simulink subsystem "PvtSubSys_HMI"  (R2020b)
settings: Solver=VariableStepAuto  StartTime=0.0  StopTime=10.0  RelTol=1e-3
undefined symbols (not defined in the file): P_HMI_LDW_LKAWarnTime, P_HMI_ObjectTypeFilter, P_HMI_WarnFormLDWReq
libraries: simulink x212, TrueDurationTime x6
(part 6 of 8)

== system PvtSubSys_HMI/HMI2.12/IFC_Signal1/Subsystem30 ==
  note: When the vehicle stops, stop updating
  note: 存在一帧丢失状况
  standstill : Inport
  in : Inport  Port=2
  Compare To Constant10 : simulink/Logic and Bit Operations/Compare To Constant  relop===  const=1  OutDataTypeStr=boolean
  Compare To Constant9 : simulink/Logic and Bit Operations/Compare To Constant  relop===  const=0  OutDataTypeStr=boolean
  Logical Operator8 : Logic  AllPortsSameDT=off  OutDataTypeStr=boolean
  MATLAB Function1 : MATLAB Function  TreatAsAtomicUnit=on
  Unit Delay : UnitDelay  SampleTime=-1  HasFrameUpgradeWarning=on
  Unit Delay3 : UnitDelay  SampleTime=-1  HasFrameUpgradeWarning=on
  out : Outport
  wires:
  Logical Operator8/1 -> MATLAB Function1/3(update)
  standstill/1 -> MATLAB Function1/1(standstill), Compare To Constant10/1, Unit Delay3/1
  Compare To Constant9/1 -> Logical Operator8/1
  in/1 -> MATLAB Function1/2(in)
  MATLAB Function1/2(recorder) -> Unit Delay/1
  Unit Delay3/1 -> Compare To Constant9/1
  Compare To Constant10/1 -> Logical Operator8/2
  Unit Delay/1 -> MATLAB Function1/4(inrecorder)
  MATLAB Function1/1(out) -> out/1

== system PvtSubSys_HMI/HMI2.12/IFC_Signal1/Subsystem31 ==
  note: 存在一帧丢失状况
  note: When the vehicle stops, stop updating
  standstill : Inport
  in : Inport  Port=2
  Compare To Constant10 : simulink/Logic and Bit Operations/Compare To Constant  relop===  const=1  OutDataTypeStr=boolean
  Compare To Constant9 : simulink/Logic and Bit Operations/Compare To Constant  relop===  const=0  OutDataTypeStr=boolean
  Logical Operator8 : Logic  AllPortsSameDT=off  OutDataTypeStr=boolean
  MATLAB Function1 : MATLAB Function  TreatAsAtomicUnit=on
  Unit Delay : UnitDelay  SampleTime=-1  HasFrameUpgradeWarning=on
  Unit Delay3 : UnitDelay  SampleTime=-1  HasFrameUpgradeWarning=on
  out : Outport
  wires:
  MATLAB Function1/1(out) -> out/1
  Unit Delay/1 -> MATLAB Function1/4(inrecorder)
  Compare To Constant10/1 -> Logical Operator8/2
  Unit Delay3/1 -> Compare To Constant9/1
  MATLAB Function1/2(recorder) -> Unit Delay/1
  in/1 -> MATLAB Function1/2(in)
  Compare To Constant9/1 -> Logical Operator8/1
  standstill/1 -> Unit Delay3/1, Compare To Constant10/1, MATLAB Function1/1(standstill)
  Logical Operator8/1 -> MATLAB Function1/3(update)

== system PvtSubSys_HMI/HMI2.12/IFC_Signal1/Subsystem32 ==
  note: When the vehicle stops, stop updating
  note: 存在一帧丢失状况
  standstill : Inport
  in : Inport  Port=2
  Compare To Constant10 : simulink/Logic and Bit Operations/Compare To Constant  relop===  const=1  OutDataTypeStr=boolean
  Compare To Constant9 : simulink/Logic and Bit Operations/Compare To Constant  relop===  const=0  OutDataTypeStr=boolean
  Logical Operator8 : Logic  AllPortsSameDT=off  OutDataTypeStr=boolean
  MATLAB Function1 : MATLAB Function  TreatAsAtomicUnit=on
  Unit Delay : UnitDelay  SampleTime=-1  HasFrameUpgradeWarning=on
  Unit Delay3 : UnitDelay  SampleTime=-1  HasFrameUpgradeWarning=on
  out : Outport
  wires:
  Logical Operator8/1 -> MATLAB Function1/3(update)
  standstill/1 -> MATLAB Function1/1(standstill), Compare To Constant10/1, Unit Delay3/1
  Compare To Constant9/1 -> Logical Operator8/1
  in/1 -> MATLAB Function1/2(in)
  MATLAB Function1/2(recorder) -> Unit Delay/1
  Unit Delay3/1 -> Compare To Constant9/1
  Compare To Constant10/1 -> Logical Operator8/2
  Unit Delay/1 -> MATLAB Function1/4(inrecorder)
  MATLAB Function1/1(out) -> out/1

== system PvtSubSys_HMI/HMI2.12/IFC_Signal1/Subsystem33 ==
  note: 存在一帧丢失状况
  note: When the vehicle stops, stop updating
  standstill : Inport
  in : Inport  Port=2
  Compare To Constant10 : simulink/Logic and Bit Operations/Compare To Constant  relop===  const=1  OutDataTypeStr=boolean
  Compare To Constant9 : simulink/Logic and Bit Operations/Compare To Constant  relop===  const=0  OutDataTypeStr=boolean
  Logical Operator8 : Logic  AllPortsSameDT=off  OutDataTypeStr=boolean
  MATLAB Function1 : MATLAB Function  TreatAsAtomicUnit=on
  Unit Delay : UnitDelay  SampleTime=-1  HasFrameUpgradeWarning=on
  Unit Delay3 : UnitDelay  SampleTime=-1  HasFrameUpgradeWarning=on
  out : Outport
  wires:
  MATLAB Function1/1(out) -> out/1
  Unit Delay/1 -> MATLAB Function1/4(inrecorder)
  Compare To Constant10/1 -> Logical Operator8/2
  Unit Delay3/1 -> Compare To Constant9/1
  MATLAB Function1/2(recorder) -> Unit Delay/1
  in/1 -> MATLAB Function1/2(in)
  Compare To Constant9/1 -> Logical Operator8/1
  standstill/1 -> Unit Delay3/1, Compare To Constant10/1, MATLAB Function1/1(standstill)
  Logical Operator8/1 -> MATLAB Function1/3(update)

== system PvtSubSys_HMI/HMI2.12/IFC_Signal1/Subsystem34 ==
  note: When the vehicle stops, stop updating
  note: 存在一帧丢失状况
  standstill : Inport
  in : Inport  Port=2
  Compare To Constant10 : simulink/Logic and Bit Operations/Compare To Constant  relop===  const=1  OutDataTypeStr=boolean
  Compare To Constant9 : simulink/Logic and Bit Operations/Compare To Constant  relop===  const=0  OutDataTypeStr=boolean
  Logical Operator8 : Logic  AllPortsSameDT=off  OutDataTypeStr=boolean
  MATLAB Function1 : MATLAB Function  TreatAsAtomicUnit=on
  Unit Delay : UnitDelay  SampleTime=-1  HasFrameUpgradeWarning=on
  Unit Delay3 : UnitDelay  SampleTime=-1  HasFrameUpgradeWarning=on
  out : Outport
  wires:
  Logical Operator8/1 -> MATLAB Function1/3(update)
  standstill/1 -> MATLAB Function1/1(standstill), Compare To Constant10/1, Unit Delay3/1
  Compare To Constant9/1 -> Logical Operator8/1
  in/1 -> MATLAB Function1/2(in)
  MATLAB Function1/2(recorder) -> Unit Delay/1
  Unit Delay3/1 -> Compare To Constant9/1
  Compare To Constant10/1 -> Logical Operator8/2
  Unit Delay/1 -> MATLAB Function1/4(inrecorder)
  MATLAB Function1/1(out) -> out/1

== system PvtSubSys_HMI/HMI2.12/IFC_Signal1/Subsystem35 ==
  note: When the vehicle stops, stop updating
  note: 存在一帧丢失状况
  standstill : Inport
  in : Inport  Port=2
  Compare To Constant10 : simulink/Logic and Bit Operations/Compare To Constant  relop===  const=1  OutDataTypeStr=boolean
  Compare To Constant9 : simulink/Logic and Bit Operations/Compare To Constant  relop===  const=0  OutDataTypeStr=boolean
  Logical Operator8 : Logic  AllPortsSameDT=off  OutDataTypeStr=boolean
  MATLAB Function1 : MATLAB Function  TreatAsAtomicUnit=on
  Unit Delay : UnitDelay  SampleTime=-1  HasFrameUpgradeWarning=on
  Unit Delay3 : UnitDelay  SampleTime=-1  HasFrameUpgradeWarning=on
  out : Outport
  wires:
  Logical Operator8/1 -> MATLAB Function1/3(update)
  standstill/1 -> MATLAB Function1/1(standstill), Compare To Constant10/1, Unit Delay3/1
  Compare To Constant9/1 -> Logical Operator8/1
  in/1 -> MATLAB Function1/2(in)
  MATLAB Function1/2(recorder) -> Unit Delay/1
  Unit Delay3/1 -> Compare To Constant9/1
  Compare To Constant10/1 -> Logical Operator8/2
  Unit Delay/1 -> MATLAB Function1/4(inrecorder)
  MATLAB Function1/1(out) -> out/1

== system PvtSubSys_HMI/HMI2.12/IFC_Signal1/Subsystem36 ==
  note: 存在一帧丢失状况
  note: When the vehicle stops, stop updating
  standstill : Inport
  in : Inport  Port=2
  Compare To Constant10 : simulink/Logic and Bit Operations/Compare To Constant  relop===  const=1  OutDataTypeStr=boolean
  Compare To Constant9 : simulink/Logic and Bit Operations/Compare To Constant  relop===  const=0  OutDataTypeStr=boolean
  Logical Operator8 : Logic  AllPortsSameDT=off  OutDataTypeStr=boolean
  MATLAB Function1 : MATLAB Function  TreatAsAtomicUnit=on
  Unit Delay : UnitDelay  SampleTime=-1  HasFrameUpgradeWarning=on
  Unit Delay3 : UnitDelay  SampleTime=-1  HasFrameUpgradeWarning=on
  out : Outport
  wires:
  MATLAB Function1/1(out) -> out/1
  Unit Delay/1 -> MATLAB Function1/4(inrecorder)
  Compare To Constant10/1 -> Logical Operator8/2
  Unit Delay3/1 -> Compare To Constant9/1
  MATLAB Function1/2(recorder) -> Unit Delay/1
  in/1 -> MATLAB Function1/2(in)
  Compare To Constant9/1 -> Logical Operator8/1
  standstill/1 -> Unit Delay3/1, Compare To Constant10/1, MATLAB Function1/1(standstill)
  Logical Operator8/1 -> MATLAB Function1/3(update)

== system PvtSubSys_HMI/HMI2.12/IFC_Signal1/Subsystem37 ==
  note: When the vehicle stops, stop updating
  note: 存在一帧丢失状况
  standstill : Inport
  in : Inport  Port=2
  Compare To Constant10 : simulink/Logic and Bit Operations/Compare To Constant  relop===  const=1  OutDataTypeStr=boolean
  Compare To Constant9 : simulink/Logic and Bit Operations/Compare To Constant  relop===  const=0  OutDataTypeStr=boolean
  Logical Operator8 : Logic  AllPortsSameDT=off  OutDataTypeStr=boolean
  MATLAB Function1 : MATLAB Function  TreatAsAtomicUnit=on
  Unit Delay : UnitDelay  SampleTime=-1  HasFrameUpgradeWarning=on
  Unit Delay3 : UnitDelay  SampleTime=-1  HasFrameUpgradeWarning=on
  out : Outport
  wires:
  Logical Operator8/1 -> MATLAB Function1/3(update)
  standstill/1 -> MATLAB Function1/1(standstill), Compare To Constant10/1, Unit Delay3/1
  Compare To Constant9/1 -> Logical Operator8/1
  in/1 -> MATLAB Function1/2(in)
  MATLAB Function1/2(recorder) -> Unit Delay/1
  Unit Delay3/1 -> Compare To Constant9/1
  Compare To Constant10/1 -> Logical Operator8/2
  Unit Delay/1 -> MATLAB Function1/4(inrecorder)
  MATLAB Function1/1(out) -> out/1

== system PvtSubSys_HMI/HMI2.12/IFC_Signal1/Subsystem38 ==
  note: 存在一帧丢失状况
  note: When the vehicle stops, stop updating
  standstill : Inport
  in : Inport  Port=2
  Compare To Constant10 : simulink/Logic and Bit Operations/Compare To Constant  relop===  const=1  OutDataTypeStr=boolean
  Compare To Constant9 : simulink/Logic and Bit Operations/Compare To Constant  relop===  const=0  OutDataTypeStr=boolean
  Logical Operator8 : Logic  AllPortsSameDT=off  OutDataTypeStr=boolean
  MATLAB Function1 : MATLAB Function  TreatAsAtomicUnit=on
  Unit Delay : UnitDelay  SampleTime=-1  HasFrameUpgradeWarning=on
  Unit Delay3 : UnitDelay  SampleTime=-1  HasFrameUpgradeWarning=on
  out : Outport
  wires:
  MATLAB Function1/1(out) -> out/1
  Unit Delay/1 -> MATLAB Function1/4(inrecorder)
  Compare To Constant10/1 -> Logical Operator8/2
  Unit Delay3/1 -> Compare To Constant9/1
  MATLAB Function1/2(recorder) -> Unit Delay/1
  in/1 -> MATLAB Function1/2(in)
  Compare To Constant9/1 -> Logical Operator8/1
  standstill/1 -> Unit Delay3/1, Compare To Constant10/1, MATLAB Function1/1(standstill)
  Logical Operator8/1 -> MATLAB Function1/3(update)

== system PvtSubSys_HMI/HMI2.12/IFC_Signal1/Subsystem39 ==
  note: When the vehicle stops, stop updating
  note: 存在一帧丢失状况
  standstill : Inport
  in : Inport  Port=2
  Compare To Constant10 : simulink/Logic and Bit Operations/Compare To Constant  relop===  const=1  OutDataTypeStr=boolean
  Compare To Constant9 : simulink/Logic and Bit Operations/Compare To Constant  relop===  const=0  OutDataTypeStr=boolean
  Logical Operator8 : Logic  AllPortsSameDT=off  OutDataTypeStr=boolean
  MATLAB Function1 : MATLAB Function  TreatAsAtomicUnit=on
  Unit Delay : UnitDelay  SampleTime=-1  HasFrameUpgradeWarning=on
  Unit Delay3 : UnitDelay  SampleTime=-1  HasFrameUpgradeWarning=on
  out : Outport
  wires:
  Logical Operator8/1 -> MATLAB Function1/3(update)
  standstill/1 -> MATLAB Function1/1(standstill), Compare To Constant10/1, Unit Delay3/1
  Compare To Constant9/1 -> Logical Operator8/1
  in/1 -> MATLAB Function1/2(in)
  MATLAB Function1/2(recorder) -> Unit Delay/1
  Unit Delay3/1 -> Compare To Constant9/1
  Compare To Constant10/1 -> Logical Operator8/2
  Unit Delay/1 -> MATLAB Function1/4(inrecorder)
  MATLAB Function1/1(out) -> out/1

== system PvtSubSys_HMI/HMI2.12/IFC_Signal1/Subsystem4 ==
  note: When the vehicle stops, stop updating
  note: 存在一帧丢失状况
  standstill : Inport
  in : Inport  Port=2
  Compare To Constant10 : simulink/Logic and Bit Operations/Compare To Constant  relop===  const=1  OutDataTypeStr=boolean
  Compare To Constant9 : simulink/Logic and Bit Operations/Compare To Constant  relop===  const=0  OutDataTypeStr=boolean
  Logical Operator8 : Logic  AllPortsSameDT=off  OutDataTypeStr=boolean
  MATLAB Function1 : MATLAB Function  TreatAsAtomicUnit=on
  Unit Delay : UnitDelay  SampleTime=-1  HasFrameUpgradeWarning=on
  Unit Delay3 : UnitDelay  SampleTime=-1  HasFrameUpgradeWarning=on
  out : Outport
  wires:
  Logical Operator8/1 -> MATLAB Function1/3(update)
  standstill/1 -> MATLAB Function1/1(standstill), Compare To Constant10/1, Unit Delay3/1
  Compare To Constant9/1 -> Logical Operator8/1
  in/1 -> MATLAB Function1/2(in)
  MATLAB Function1/2(recorder) -> Unit Delay/1
  Unit Delay3/1 -> Compare To Constant9/1
  Compare To Constant10/1 -> Logical Operator8/2
  Unit Delay/1 -> MATLAB Function1/4(inrecorder)
  MATLAB Function1/1(out) -> out/1

== system PvtSubSys_HMI/HMI2.12/IFC_Signal1/Subsystem40 ==
  note: 存在一帧丢失状况
  note: When the vehicle stops, stop updating
  standstill : Inport
  in : Inport  Port=2
  Compare To Constant10 : simulink/Logic and Bit Operations/Compare To Constant  relop===  const=1  OutDataTypeStr=boolean
  Compare To Constant9 : simulink/Logic and Bit Operations/Compare To Constant  relop===  const=0  OutDataTypeStr=boolean
  Logical Operator8 : Logic  AllPortsSameDT=off  OutDataTypeStr=boolean
  MATLAB Function1 : MATLAB Function  TreatAsAtomicUnit=on
  Unit Delay : UnitDelay  SampleTime=-1  HasFrameUpgradeWarning=on
  Unit Delay3 : UnitDelay  SampleTime=-1  HasFrameUpgradeWarning=on
  out : Outport
  wires:
  MATLAB Function1/1(out) -> out/1
  Unit Delay/1 -> MATLAB Function1/4(inrecorder)
  Compare To Constant10/1 -> Logical Operator8/2
  Unit Delay3/1 -> Compare To Constant9/1
  MATLAB Function1/2(recorder) -> Unit Delay/1
  in/1 -> MATLAB Function1/2(in)
  Compare To Constant9/1 -> Logical Operator8/1
  standstill/1 -> Unit Delay3/1, Compare To Constant10/1, MATLAB Function1/1(standstill)
  Logical Operator8/1 -> MATLAB Function1/3(update)

== system PvtSubSys_HMI/HMI2.12/IFC_Signal1/Subsystem41 ==
  note: 存在一帧丢失状况
  note: When the vehicle stops, stop updating
  standstill : Inport
  in : Inport  Port=2
  Compare To Constant10 : simulink/Logic and Bit Operations/Compare To Constant  relop===  const=1  OutDataTypeStr=boolean
  Compare To Constant9 : simulink/Logic and Bit Operations/Compare To Constant  relop===  const=0  OutDataTypeStr=boolean
  Logical Operator8 : Logic  AllPortsSameDT=off  OutDataTypeStr=boolean
  MATLAB Function1 : MATLAB Function  TreatAsAtomicUnit=on
  Unit Delay : UnitDelay  SampleTime=-1  HasFrameUpgradeWarning=on
  Unit Delay3 : UnitDelay  SampleTime=-1  HasFrameUpgradeWarning=on
  out : Outport
  wires:
  MATLAB Function1/1(out) -> out/1
  Unit Delay/1 -> MATLAB Function1/4(inrecorder)
  Compare To Constant10/1 -> Logical Operator8/2
  Unit Delay3/1 -> Compare To Constant9/1
  MATLAB Function1/2(recorder) -> Unit Delay/1
  in/1 -> MATLAB Function1/2(in)
  Compare To Constant9/1 -> Logical Operator8/1
  standstill/1 -> Unit Delay3/1, Compare To Constant10/1, MATLAB Function1/1(standstill)
  Logical Operator8/1 -> MATLAB Function1/3(update)

== system PvtSubSys_HMI/HMI2.12/IFC_Signal1/Subsystem42 ==
  note: When the vehicle stops, stop updating
  note: 存在一帧丢失状况
  standstill : Inport
  in : Inport  Port=2
  Compare To Constant10 : simulink/Logic and Bit Operations/Compare To Constant  relop===  const=1  OutDataTypeStr=boolean
  Compare To Constant9 : simulink/Logic and Bit Operations/Compare To Constant  relop===  const=0  OutDataTypeStr=boolean
  Logical Operator8 : Logic  AllPortsSameDT=off  OutDataTypeStr=boolean
  MATLAB Function1 : MATLAB Function  TreatAsAtomicUnit=on
  Unit Delay : UnitDelay  SampleTime=-1  HasFrameUpgradeWarning=on
  Unit Delay3 : UnitDelay  SampleTime=-1  HasFrameUpgradeWarning=on
  out : Outport
  wires:
  Logical Operator8/1 -> MATLAB Function1/3(update)
  standstill/1 -> MATLAB Function1/1(standstill), Compare To Constant10/1, Unit Delay3/1
  Compare To Constant9/1 -> Logical Operator8/1
  in/1 -> MATLAB Function1/2(in)
  MATLAB Function1/2(recorder) -> Unit Delay/1
  Unit Delay3/1 -> Compare To Constant9/1
  Compare To Constant10/1 -> Logical Operator8/2
  Unit Delay/1 -> MATLAB Function1/4(inrecorder)
  MATLAB Function1/1(out) -> out/1

== system PvtSubSys_HMI/HMI2.12/IFC_Signal1/Subsystem43 ==
  note: 存在一帧丢失状况
  note: When the vehicle stops, stop updating
  standstill : Inport
  in : Inport  Port=2
  Compare To Constant10 : simulink/Logic and Bit Operations/Compare To Constant  relop===  const=1  OutDataTypeStr=boolean
  Compare To Constant9 : simulink/Logic and Bit Operations/Compare To Constant  relop===  const=0  OutDataTypeStr=boolean
  Logical Operator8 : Logic  AllPortsSameDT=off  OutDataTypeStr=boolean
  MATLAB Function1 : MATLAB Function  TreatAsAtomicUnit=on
  Unit Delay : UnitDelay  SampleTime=-1  HasFrameUpgradeWarning=on
  Unit Delay3 : UnitDelay  SampleTime=-1  HasFrameUpgradeWarning=on
  out : Outport
  wires:
  MATLAB Function1/1(out) -> out/1
  Unit Delay/1 -> MATLAB Function1/4(inrecorder)
  Compare To Constant10/1 -> Logical Operator8/2
  Unit Delay3/1 -> Compare To Constant9/1
  MATLAB Function1/2(recorder) -> Unit Delay/1
  in/1 -> MATLAB Function1/2(in)
  Compare To Constant9/1 -> Logical Operator8/1
  standstill/1 -> Unit Delay3/1, Compare To Constant10/1, MATLAB Function1/1(standstill)
  Logical Operator8/1 -> MATLAB Function1/3(update)

== system PvtSubSys_HMI/HMI2.12/IFC_Signal1/Subsystem44 ==
  note: When the vehicle stops, stop updating
  note: 存在一帧丢失状况
  standstill : Inport
  in : Inport  Port=2
  Compare To Constant10 : simulink/Logic and Bit Operations/Compare To Constant  relop===  const=1  OutDataTypeStr=boolean
  Compare To Constant9 : simulink/Logic and Bit Operations/Compare To Constant  relop===  const=0  OutDataTypeStr=boolean
  Logical Operator8 : Logic  AllPortsSameDT=off  OutDataTypeStr=boolean
  MATLAB Function1 : MATLAB Function  TreatAsAtomicUnit=on
  Unit Delay : UnitDelay  SampleTime=-1  HasFrameUpgradeWarning=on
  Unit Delay3 : UnitDelay  SampleTime=-1  HasFrameUpgradeWarning=on
  out : Outport
  wires:
  Logical Operator8/1 -> MATLAB Function1/3(update)
  standstill/1 -> MATLAB Function1/1(standstill), Compare To Constant10/1, Unit Delay3/1
  Compare To Constant9/1 -> Logical Operator8/1
  in/1 -> MATLAB Function1/2(in)
  MATLAB Function1/2(recorder) -> Unit Delay/1
  Unit Delay3/1 -> Compare To Constant9/1
  Compare To Constant10/1 -> Logical Operator8/2
  Unit Delay/1 -> MATLAB Function1/4(inrecorder)
  MATLAB Function1/1(out) -> out/1

== system PvtSubSys_HMI/HMI2.12/IFC_Signal1/Subsystem45 ==
  note: 存在一帧丢失状况
  note: When the vehicle stops, stop updating
  standstill : Inport
  in : Inport  Port=2
  Compare To Constant10 : simulink/Logic and Bit Operations/Compare To Constant  relop===  const=1  OutDataTypeStr=boolean
  Compare To Constant9 : simulink/Logic and Bit Operations/Compare To Constant  relop===  const=0  OutDataTypeStr=boolean
  Logical Operator8 : Logic  AllPortsSameDT=off  OutDataTypeStr=boolean
  MATLAB Function1 : MATLAB Function  TreatAsAtomicUnit=on
  Unit Delay : UnitDelay  SampleTime=-1  HasFrameUpgradeWarning=on
  Unit Delay3 : UnitDelay  SampleTime=-1  HasFrameUpgradeWarning=on
  out : Outport
  wires:
  MATLAB Function1/1(out) -> out/1
  Unit Delay/1 -> MATLAB Function1/4(inrecorder)
  Compare To Constant10/1 -> Logical Operator8/2
  Unit Delay3/1 -> Compare To Constant9/1
  MATLAB Function1/2(recorder) -> Unit Delay/1
  in/1 -> MATLAB Function1/2(in)
  Compare To Constant9/1 -> Logical Operator8/1
  standstill/1 -> Unit Delay3/1, Compare To Constant10/1, MATLAB Function1/1(standstill)
  Logical Operator8/1 -> MATLAB Function1/3(update)

== system PvtSubSys_HMI/HMI2.12/IFC_Signal1/Subsystem46 ==
  note: When the vehicle stops, stop updating
  note: 存在一帧丢失状况
  standstill : Inport
  in : Inport  Port=2
  Compare To Constant10 : simulink/Logic and Bit Operations/Compare To Constant  relop===  const=1  OutDataTypeStr=boolean
  Compare To Constant9 : simulink/Logic and Bit Operations/Compare To Constant  relop===  const=0  OutDataTypeStr=boolean
  Logical Operator8 : Logic  AllPortsSameDT=off  OutDataTypeStr=boolean
  MATLAB Function1 : MATLAB Function  TreatAsAtomicUnit=on
  Unit Delay : UnitDelay  SampleTime=-1  HasFrameUpgradeWarning=on
  Unit Delay3 : UnitDelay  SampleTime=-1  HasFrameUpgradeWarning=on
  out : Outport
  wires:
  Logical Operator8/1 -> MATLAB Function1/3(update)
  standstill/1 -> MATLAB Function1/1(standstill), Compare To Constant10/1, Unit Delay3/1
  Compare To Constant9/1 -> Logical Operator8/1
  in/1 -> MATLAB Function1/2(in)
  MATLAB Function1/2(recorder) -> Unit Delay/1
  Unit Delay3/1 -> Compare To Constant9/1
  Compare To Constant10/1 -> Logical Operator8/2
  Unit Delay/1 -> MATLAB Function1/4(inrecorder)
  MATLAB Function1/1(out) -> out/1

== system PvtSubSys_HMI/HMI2.12/IFC_Signal1/Subsystem47 ==
  note: 存在一帧丢失状况
  note: When the vehicle stops, stop updating
  standstill : Inport
  in : Inport  Port=2
  Compare To Constant10 : simulink/Logic and Bit Operations/Compare To Constant  relop===  const=1  OutDataTypeStr=boolean
  Compare To Constant9 : simulink/Logic and Bit Operations/Compare To Constant  relop===  const=0  OutDataTypeStr=boolean
  Logical Operator8 : Logic  AllPortsSameDT=off  OutDataTypeStr=boolean
  MATLAB Function1 : MATLAB Function  TreatAsAtomicUnit=on
  Unit Delay : UnitDelay  SampleTime=-1  HasFrameUpgradeWarning=on
  Unit Delay3 : UnitDelay  SampleTime=-1  HasFrameUpgradeWarning=on
  out : Outport
  wires:
  MATLAB Function1/1(out) -> out/1
  Unit Delay/1 -> MATLAB Function1/4(inrecorder)
  Compare To Constant10/1 -> Logical Operator8/2
  Unit Delay3/1 -> Compare To Constant9/1
  MATLAB Function1/2(recorder) -> Unit Delay/1
  in/1 -> MATLAB Function1/2(in)
  Compare To Constant9/1 -> Logical Operator8/1
  standstill/1 -> Unit Delay3/1, Compare To Constant10/1, MATLAB Function1/1(standstill)
  Logical Operator8/1 -> MATLAB Function1/3(update)

== system PvtSubSys_HMI/HMI2.12/IFC_Signal1/Subsystem48 ==
  note: When the vehicle stops, stop updating
  note: 存在一帧丢失状况
  standstill : Inport
  in : Inport  Port=2
  Compare To Constant10 : simulink/Logic and Bit Operations/Compare To Constant  relop===  const=1  OutDataTypeStr=boolean
  Compare To Constant9 : simulink/Logic and Bit Operations/Compare To Constant  relop===  const=0  OutDataTypeStr=boolean
  Logical Operator8 : Logic  AllPortsSameDT=off  OutDataTypeStr=boolean
  MATLAB Function1 : MATLAB Function  TreatAsAtomicUnit=on
  Unit Delay : UnitDelay  SampleTime=-1  HasFrameUpgradeWarning=on
  Unit Delay3 : UnitDelay  SampleTime=-1  HasFrameUpgradeWarning=on
  out : Outport
  wires:
  Logical Operator8/1 -> MATLAB Function1/3(update)
  standstill/1 -> MATLAB Function1/1(standstill), Compare To Constant10/1, Unit Delay3/1
  Compare To Constant9/1 -> Logical Operator8/1
  in/1 -> MATLAB Function1/2(in)
  MATLAB Function1/2(recorder) -> Unit Delay/1
  Unit Delay3/1 -> Compare To Constant9/1
  Compare To Constant10/1 -> Logical Operator8/2
  Unit Delay/1 -> MATLAB Function1/4(inrecorder)
  MATLAB Function1/1(out) -> out/1

== system PvtSubSys_HMI/HMI2.12/IFC_Signal1/Subsystem49 ==
  note: 存在一帧丢失状况
  note: When the vehicle stops, stop updating
  standstill : Inport
  in : Inport  Port=2
  Compare To Constant10 : simulink/Logic and Bit Operations/Compare To Constant  relop===  const=1  OutDataTypeStr=boolean
  Compare To Constant9 : simulink/Logic and Bit Operations/Compare To Constant  relop===  const=0  OutDataTypeStr=boolean
  Logical Operator8 : Logic  AllPortsSameDT=off  OutDataTypeStr=boolean
  MATLAB Function1 : MATLAB Function  TreatAsAtomicUnit=on
  Unit Delay : UnitDelay  SampleTime=-1  HasFrameUpgradeWarning=on
  Unit Delay3 : UnitDelay  SampleTime=-1  HasFrameUpgradeWarning=on
  out : Outport
  wires:
  MATLAB Function1/1(out) -> out/1
  Unit Delay/1 -> MATLAB Function1/4(inrecorder)
  Compare To Constant10/1 -> Logical Operator8/2
  Unit Delay3/1 -> Compare To Constant9/1
  MATLAB Function1/2(recorder) -> Unit Delay/1
  in/1 -> MATLAB Function1/2(in)
  Compare To Constant9/1 -> Logical Operator8/1
  standstill/1 -> Unit Delay3/1, Compare To Constant10/1, MATLAB Function1/1(standstill)
  Logical Operator8/1 -> MATLAB Function1/3(update)

== system PvtSubSys_HMI/HMI2.12/IFC_Signal1/Subsystem5 ==
  note: 存在一帧丢失状况
  note: When the vehicle stops, stop updating
  standstill : Inport
  in : Inport  Port=2
  Compare To Constant10 : simulink/Logic and Bit Operations/Compare To Constant  relop===  const=1  OutDataTypeStr=boolean
  Compare To Constant9 : simulink/Logic and Bit Operations/Compare To Constant  relop===  const=0  OutDataTypeStr=boolean
  Logical Operator8 : Logic  AllPortsSameDT=off  OutDataTypeStr=boolean
  MATLAB Function1 : MATLAB Function  TreatAsAtomicUnit=on
  Unit Delay : UnitDelay  SampleTime=-1  HasFrameUpgradeWarning=on
  Unit Delay3 : UnitDelay  SampleTime=-1  HasFrameUpgradeWarning=on
  out : Outport
  wires:
  MATLAB Function1/1(out) -> out/1
  Unit Delay/1 -> MATLAB Function1/4(inrecorder)
  Compare To Constant10/1 -> Logical Operator8/2
  Unit Delay3/1 -> Compare To Constant9/1
  MATLAB Function1/2(recorder) -> Unit Delay/1
  in/1 -> MATLAB Function1/2(in)
  Compare To Constant9/1 -> Logical Operator8/1
  standstill/1 -> Unit Delay3/1, Compare To Constant10/1, MATLAB Function1/1(standstill)
  Logical Operator8/1 -> MATLAB Function1/3(update)

== system PvtSubSys_HMI/HMI2.12/IFC_Signal1/Subsystem50 ==
  note: When the vehicle stops, stop updating
  note: 存在一帧丢失状况
  standstill : Inport
  in : Inport  Port=2
  Compare To Constant10 : simulink/Logic and Bit Operations/Compare To Constant  relop===  const=1  OutDataTypeStr=boolean
  Compare To Constant9 : simulink/Logic and Bit Operations/Compare To Constant  relop===  const=0  OutDataTypeStr=boolean
  Logical Operator8 : Logic  AllPortsSameDT=off  OutDataTypeStr=boolean
  MATLAB Function1 : MATLAB Function  TreatAsAtomicUnit=on
  Unit Delay : UnitDelay  SampleTime=-1  HasFrameUpgradeWarning=on
  Unit Delay3 : UnitDelay  SampleTime=-1  HasFrameUpgradeWarning=on
  out : Outport
  wires:
  Logical Operator8/1 -> MATLAB Function1/3(update)
  standstill/1 -> MATLAB Function1/1(standstill), Compare To Constant10/1, Unit Delay3/1
  Compare To Constant9/1 -> Logical Operator8/1
  in/1 -> MATLAB Function1/2(in)
  MATLAB Function1/2(recorder) -> Unit Delay/1
  Unit Delay3/1 -> Compare To Constant9/1
  Compare To Constant10/1 -> Logical Operator8/2
  Unit Delay/1 -> MATLAB Function1/4(inrecorder)
  MATLAB Function1/1(out) -> out/1

== system PvtSubSys_HMI/HMI2.12/IFC_Signal1/Subsystem51 ==
  note: 存在一帧丢失状况
  note: When the vehicle stops, stop updating
  standstill : Inport
  in : Inport  Port=2
  Compare To Constant10 : simulink/Logic and Bit Operations/Compare To Constant  relop===  const=1  OutDataTypeStr=boolean
  Compare To Constant9 : simulink/Logic and Bit Operations/Compare To Constant  relop===  const=0  OutDataTypeStr=boolean
  Logical Operator8 : Logic  AllPortsSameDT=off  OutDataTypeStr=boolean
  MATLAB Function1 : MATLAB Function  TreatAsAtomicUnit=on
  Unit Delay : UnitDelay  SampleTime=-1  HasFrameUpgradeWarning=on
  Unit Delay3 : UnitDelay  SampleTime=-1  HasFrameUpgradeWarning=on
  out : Outport
  wires:
  MATLAB Function1/1(out) -> out/1
  Unit Delay/1 -> MATLAB Function1/4(inrecorder)
  Compare To Constant10/1 -> Logical Operator8/2
  Unit Delay3/1 -> Compare To Constant9/1
  MATLAB Function1/2(recorder) -> Unit Delay/1
  in/1 -> MATLAB Function1/2(in)
  Compare To Constant9/1 -> Logical Operator8/1
  standstill/1 -> Unit Delay3/1, Compare To Constant10/1, MATLAB Function1/1(standstill)
  Logical Operator8/1 -> MATLAB Function1/3(update)

== system PvtSubSys_HMI/HMI2.12/IFC_Signal1/Subsystem52 ==
  note: When the vehicle stops, stop updating
  note: 存在一帧丢失状况
  standstill : Inport
  in : Inport  Port=2
  Compare To Constant10 : simulink/Logic and Bit Operations/Compare To Constant  relop===  const=1  OutDataTypeStr=boolean
  Compare To Constant9 : simulink/Logic and Bit Operations/Compare To Constant  relop===  const=0  OutDataTypeStr=boolean
  Logical Operator8 : Logic  AllPortsSameDT=off  OutDataTypeStr=boolean
  MATLAB Function1 : MATLAB Function  TreatAsAtomicUnit=on
  Unit Delay : UnitDelay  SampleTime=-1  HasFrameUpgradeWarning=on
  Unit Delay3 : UnitDelay  SampleTime=-1  HasFrameUpgradeWarning=on
  out : Outport
  wires:
  Logical Operator8/1 -> MATLAB Function1/3(update)
  standstill/1 -> MATLAB Function1/1(standstill), Compare To Constant10/1, Unit Delay3/1
  Compare To Constant9/1 -> Logical Operator8/1
  in/1 -> MATLAB Function1/2(in)
  MATLAB Function1/2(recorder) -> Unit Delay/1
  Unit Delay3/1 -> Compare To Constant9/1
  Compare To Constant10/1 -> Logical Operator8/2
  Unit Delay/1 -> MATLAB Function1/4(inrecorder)
  MATLAB Function1/1(out) -> out/1

== system PvtSubSys_HMI/HMI2.12/IFC_Signal1/Subsystem53 ==
  note: 存在一帧丢失状况
  note: When the vehicle stops, stop updating
  standstill : Inport
  in : Inport  Port=2
  Compare To Constant10 : simulink/Logic and Bit Operations/Compare To Constant  relop===  const=1  OutDataTypeStr=boolean
  Compare To Constant9 : simulink/Logic and Bit Operations/Compare To Constant  relop===  const=0  OutDataTypeStr=boolean
  Logical Operator8 : Logic  AllPortsSameDT=off  OutDataTypeStr=boolean
  MATLAB Function1 : MATLAB Function  TreatAsAtomicUnit=on
  Unit Delay : UnitDelay  SampleTime=-1  HasFrameUpgradeWarning=on
  Unit Delay3 : UnitDelay  SampleTime=-1  HasFrameUpgradeWarning=on
  out : Outport
  wires:
  MATLAB Function1/1(out) -> out/1
  Unit Delay/1 -> MATLAB Function1/4(inrecorder)
  Compare To Constant10/1 -> Logical Operator8/2
  Unit Delay3/1 -> Compare To Constant9/1
  MATLAB Function1/2(recorder) -> Unit Delay/1
  in/1 -> MATLAB Function1/2(in)
  Compare To Constant9/1 -> Logical Operator8/1
  standstill/1 -> Unit Delay3/1, Compare To Constant10/1, MATLAB Function1/1(standstill)
  Logical Operator8/1 -> MATLAB Function1/3(update)

== system PvtSubSys_HMI/HMI2.12/IFC_Signal1/Subsystem54 ==
  note: 存在一帧丢失状况
  note: When the vehicle stops, stop updating
  standstill : Inport
  in : Inport  Port=2
  Compare To Constant10 : simulink/Logic and Bit Operations/Compare To Constant  relop===  const=1  OutDataTypeStr=boolean
  Compare To Constant9 : simulink/Logic and Bit Operations/Compare To Constant  relop===  const=0  OutDataTypeStr=boolean
  Logical Operator8 : Logic  AllPortsSameDT=off  OutDataTypeStr=boolean
  MATLAB Function1 : MATLAB Function  TreatAsAtomicUnit=on
  Unit Delay : UnitDelay  SampleTime=-1  HasFrameUpgradeWarning=on
  Unit Delay3 : UnitDelay  SampleTime=-1  HasFrameUpgradeWarning=on
  out : Outport
  wires:
  MATLAB Function1/1(out) -> out/1
  Unit Delay/1 -> MATLAB Function1/4(inrecorder)
  Compare To Constant10/1 -> Logical Operator8/2
  Unit Delay3/1 -> Compare To Constant9/1
  MATLAB Function1/2(recorder) -> Unit Delay/1
  in/1 -> MATLAB Function1/2(in)
  Compare To Constant9/1 -> Logical Operator8/1
  standstill/1 -> Unit Delay3/1, Compare To Constant10/1, MATLAB Function1/1(standstill)
  Logical Operator8/1 -> MATLAB Function1/3(update)

== system PvtSubSys_HMI/HMI2.12/IFC_Signal1/Subsystem55 ==
  note: When the vehicle stops, stop updating
  note: 存在一帧丢失状况
  standstill : Inport
  in : Inport  Port=2
  Compare To Constant10 : simulink/Logic and Bit Operations/Compare To Constant  relop===  const=1  OutDataTypeStr=boolean
  Compare To Constant9 : simulink/Logic and Bit Operations/Compare To Constant  relop===  const=0  OutDataTypeStr=boolean
  Logical Operator8 : Logic  AllPortsSameDT=off  OutDataTypeStr=boolean
  MATLAB Function1 : MATLAB Function  TreatAsAtomicUnit=on
  Unit Delay : UnitDelay  SampleTime=-1  HasFrameUpgradeWarning=on
  Unit Delay3 : UnitDelay  SampleTime=-1  HasFrameUpgradeWarning=on
  out : Outport
  wires:
  Logical Operator8/1 -> MATLAB Function1/3(update)
  standstill/1 -> MATLAB Function1/1(standstill), Compare To Constant10/1, Unit Delay3/1
  Compare To Constant9/1 -> Logical Operator8/1
  in/1 -> MATLAB Function1/2(in)
  MATLAB Function1/2(recorder) -> Unit Delay/1
  Unit Delay3/1 -> Compare To Constant9/1
  Compare To Constant10/1 -> Logical Operator8/2
  Unit Delay/1 -> MATLAB Function1/4(inrecorder)
  MATLAB Function1/1(out) -> out/1

== system PvtSubSys_HMI/HMI2.12/IFC_Signal1/Subsystem56 ==
  note: 存在一帧丢失状况
  note: When the vehicle stops, stop updating
  standstill : Inport
  in : Inport  Port=2
  Compare To Constant10 : simulink/Logic and Bit Operations/Compare To Constant  relop===  const=1  OutDataTypeStr=boolean
  Compare To Constant9 : simulink/Logic and Bit Operations/Compare To Constant  relop===  const=0  OutDataTypeStr=boolean
  Logical Operator8 : Logic  AllPortsSameDT=off  OutDataTypeStr=boolean
  MATLAB Function1 : MATLAB Function  TreatAsAtomicUnit=on
  Unit Delay : UnitDelay  SampleTime=-1  HasFrameUpgradeWarning=on
  Unit Delay3 : UnitDelay  SampleTime=-1  HasFrameUpgradeWarning=on
  out : Outport
  wires:
  MATLAB Function1/1(out) -> out/1
  Unit Delay/1 -> MATLAB Function1/4(inrecorder)
  Compare To Constant10/1 -> Logical Operator8/2
  Unit Delay3/1 -> Compare To Constant9/1
  MATLAB Function1/2(recorder) -> Unit Delay/1
  in/1 -> MATLAB Function1/2(in)
  Compare To Constant9/1 -> Logical Operator8/1
  standstill/1 -> Unit Delay3/1, Compare To Constant10/1, MATLAB Function1/1(standstill)
  Logical Operator8/1 -> MATLAB Function1/3(update)

== system PvtSubSys_HMI/HMI2.12/IFC_Signal1/Subsystem57 ==
  note: When the vehicle stops, stop updating
  note: 存在一帧丢失状况
  standstill : Inport
  in : Inport  Port=2
  Compare To Constant10 : simulink/Logic and Bit Operations/Compare To Constant  relop===  const=1  OutDataTypeStr=boolean
  Compare To Constant9 : simulink/Logic and Bit Operations/Compare To Constant  relop===  const=0  OutDataTypeStr=boolean
  Logical Operator8 : Logic  AllPortsSameDT=off  OutDataTypeStr=boolean
  MATLAB Function1 : MATLAB Function  TreatAsAtomicUnit=on
  Unit Delay : UnitDelay  SampleTime=-1  HasFrameUpgradeWarning=on
  Unit Delay3 : UnitDelay  SampleTime=-1  HasFrameUpgradeWarning=on
  out : Outport
  wires:
  Logical Operator8/1 -> MATLAB Function1/3(update)
  standstill/1 -> MATLAB Function1/1(standstill), Compare To Constant10/1, Unit Delay3/1
  Compare To Constant9/1 -> Logical Operator8/1
  in/1 -> MATLAB Function1/2(in)
  MATLAB Function1/2(recorder) -> Unit Delay/1
  Unit Delay3/1 -> Compare To Constant9/1
  Compare To Constant10/1 -> Logical Operator8/2
  Unit Delay/1 -> MATLAB Function1/4(inrecorder)
  MATLAB Function1/1(out) -> out/1

== system PvtSubSys_HMI/HMI2.12/IFC_Signal1/Subsystem58 ==
  note: 存在一帧丢失状况
  note: When the vehicle stops, stop updating
  standstill : Inport
  in : Inport  Port=2
  Compare To Constant10 : simulink/Logic and Bit Operations/Compare To Constant  relop===  const=1  OutDataTypeStr=boolean
  Compare To Constant9 : simulink/Logic and Bit Operations/Compare To Constant  relop===  const=0  OutDataTypeStr=boolean
  Logical Operator8 : Logic  AllPortsSameDT=off  OutDataTypeStr=boolean
  MATLAB Function1 : MATLAB Function  TreatAsAtomicUnit=on
  Unit Delay : UnitDelay  SampleTime=-1  HasFrameUpgradeWarning=on
  Unit Delay3 : UnitDelay  SampleTime=-1  HasFrameUpgradeWarning=on
  out : Outport
  wires:
  MATLAB Function1/1(out) -> out/1
  Unit Delay/1 -> MATLAB Function1/4(inrecorder)
  Compare To Constant10/1 -> Logical Operator8/2
  Unit Delay3/1 -> Compare To Constant9/1
  MATLAB Function1/2(recorder) -> Unit Delay/1
  in/1 -> MATLAB Function1/2(in)
  Compare To Constant9/1 -> Logical Operator8/1
  standstill/1 -> Unit Delay3/1, Compare To Constant10/1, MATLAB Function1/1(standstill)
  Logical Operator8/1 -> MATLAB Function1/3(update)

== system PvtSubSys_HMI/HMI2.12/IFC_Signal1/Subsystem59 ==
  note: 存在一帧丢失状况
  note: When the vehicle stops, stop updating
  standstill : Inport
  in : Inport  Port=2
  Compare To Constant10 : simulink/Logic and Bit Operations/Compare To Constant  relop===  const=1  OutDataTypeStr=boolean
  Compare To Constant9 : simulink/Logic and Bit Operations/Compare To Constant  relop===  const=0  OutDataTypeStr=boolean
  Logical Operator8 : Logic  AllPortsSameDT=off  OutDataTypeStr=boolean
  MATLAB Function1 : MATLAB Function  TreatAsAtomicUnit=on
  Unit Delay : UnitDelay  SampleTime=-1  HasFrameUpgradeWarning=on
  Unit Delay3 : UnitDelay  SampleTime=-1  HasFrameUpgradeWarning=on
  out : Outport
  wires:
  MATLAB Function1/1(out) -> out/1
  Unit Delay/1 -> MATLAB Function1/4(inrecorder)
  Compare To Constant10/1 -> Logical Operator8/2
  Unit Delay3/1 -> Compare To Constant9/1
  MATLAB Function1/2(recorder) -> Unit Delay/1
  in/1 -> MATLAB Function1/2(in)
  Compare To Constant9/1 -> Logical Operator8/1
  standstill/1 -> Unit Delay3/1, Compare To Constant10/1, MATLAB Function1/1(standstill)
  Logical Operator8/1 -> MATLAB Function1/3(update)

== system PvtSubSys_HMI/HMI2.12/IFC_Signal1/Subsystem6 ==
  note: When the vehicle stops, stop updating
  note: 存在一帧丢失状况
  standstill : Inport
  in : Inport  Port=2
  Compare To Constant10 : simulink/Logic and Bit Operations/Compare To Constant  relop===  const=1  OutDataTypeStr=boolean
  Compare To Constant9 : simulink/Logic and Bit Operations/Compare To Constant  relop===  const=0  OutDataTypeStr=boolean
  Logical Operator8 : Logic  AllPortsSameDT=off  OutDataTypeStr=boolean
  MATLAB Function1 : MATLAB Function  TreatAsAtomicUnit=on
  Unit Delay : UnitDelay  SampleTime=-1  HasFrameUpgradeWarning=on
  Unit Delay3 : UnitDelay  SampleTime=-1  HasFrameUpgradeWarning=on
  out : Outport
  wires:
  Logical Operator8/1 -> MATLAB Function1/3(update)
  standstill/1 -> MATLAB Function1/1(standstill), Compare To Constant10/1, Unit Delay3/1
  Compare To Constant9/1 -> Logical Operator8/1
  in/1 -> MATLAB Function1/2(in)
  MATLAB Function1/2(recorder) -> Unit Delay/1
  Unit Delay3/1 -> Compare To Constant9/1
  Compare To Constant10/1 -> Logical Operator8/2
  Unit Delay/1 -> MATLAB Function1/4(inrecorder)
  MATLAB Function1/1(out) -> out/1

== system PvtSubSys_HMI/HMI2.12/IFC_Signal1/Subsystem7 ==
  note: 存在一帧丢失状况
  note: When the vehicle stops, stop updating
  standstill : Inport
  in : Inport  Port=2
  Compare To Constant10 : simulink/Logic and Bit Operations/Compare To Constant  relop===  const=1  OutDataTypeStr=boolean
  Compare To Constant9 : simulink/Logic and Bit Operations/Compare To Constant  relop===  const=0  OutDataTypeStr=boolean
  Logical Operator8 : Logic  AllPortsSameDT=off  OutDataTypeStr=boolean
  MATLAB Function1 : MATLAB Function  TreatAsAtomicUnit=on
  Unit Delay : UnitDelay  SampleTime=-1  HasFrameUpgradeWarning=on
  Unit Delay3 : UnitDelay  SampleTime=-1  HasFrameUpgradeWarning=on
  out : Outport
  wires:
  MATLAB Function1/1(out) -> out/1
  Unit Delay/1 -> MATLAB Function1/4(inrecorder)
  Compare To Constant10/1 -> Logical Operator8/2
  Unit Delay3/1 -> Compare To Constant9/1
  MATLAB Function1/2(recorder) -> Unit Delay/1
  in/1 -> MATLAB Function1/2(in)
  Compare To Constant9/1 -> Logical Operator8/1
  standstill/1 -> Unit Delay3/1, Compare To Constant10/1, MATLAB Function1/1(standstill)
  Logical Operator8/1 -> MATLAB Function1/3(update)

== system PvtSubSys_HMI/HMI2.12/IFC_Signal1/Subsystem8 ==
  note: When the vehicle stops, stop updating
  note: 存在一帧丢失状况
  standstill : Inport
  in : Inport  Port=2
  Compare To Constant10 : simulink/Logic and Bit Operations/Compare To Constant  relop===  const=1  OutDataTypeStr=boolean
  Compare To Constant9 : simulink/Logic and Bit Operations/Compare To Constant  relop===  const=0  OutDataTypeStr=boolean
  Logical Operator8 : Logic  AllPortsSameDT=off  OutDataTypeStr=boolean
  MATLAB Function1 : MATLAB Function  TreatAsAtomicUnit=on
  Unit Delay : UnitDelay  SampleTime=-1  HasFrameUpgradeWarning=on
  Unit Delay3 : UnitDelay  SampleTime=-1  HasFrameUpgradeWarning=on
  out : Outport
  wires:
  Logical Operator8/1 -> MATLAB Function1/3(update)
  standstill/1 -> MATLAB Function1/1(standstill), Compare To Constant10/1, Unit Delay3/1
  Compare To Constant9/1 -> Logical Operator8/1
  in/1 -> MATLAB Function1/2(in)
  MATLAB Function1/2(recorder) -> Unit Delay/1
  Unit Delay3/1 -> Compare To Constant9/1
  Compare To Constant10/1 -> Logical Operator8/2
  Unit Delay/1 -> MATLAB Function1/4(inrecorder)
  MATLAB Function1/1(out) -> out/1

== system PvtSubSys_HMI/HMI2.12/IFC_Signal1/Subsystem9 ==
  note: 存在一帧丢失状况
  note: When the vehicle stops, stop updating
  standstill : Inport
  in : Inport  Port=2
  Compare To Constant10 : simulink/Logic and Bit Operations/Compare To Constant  relop===  const=1  OutDataTypeStr=boolean
  Compare To Constant9 : simulink/Logic and Bit Operations/Compare To Constant  relop===  const=0  OutDataTypeStr=boolean
  Logical Operator8 : Logic  AllPortsSameDT=off  OutDataTypeStr=boolean
  MATLAB Function1 : MATLAB Function  TreatAsAtomicUnit=on
  Unit Delay : UnitDelay  SampleTime=-1  HasFrameUpgradeWarning=on
  Unit Delay3 : UnitDelay  SampleTime=-1  HasFrameUpgradeWarning=on
  out : Outport
  wires:
  MATLAB Function1/1(out) -> out/1
  Unit Delay/1 -> MATLAB Function1/4(inrecorder)
  Compare To Constant10/1 -> Logical Operator8/2
  Unit Delay3/1 -> Compare To Constant9/1
  MATLAB Function1/2(recorder) -> Unit Delay/1
  in/1 -> MATLAB Function1/2(in)
  Compare To Constant9/1 -> Logical Operator8/1
  standstill/1 -> Unit Delay3/1, Compare To Constant10/1, MATLAB Function1/1(standstill)
  Logical Operator8/1 -> MATLAB Function1/3(update)

== system PvtSubSys_HMI/HMI2.12/IFC_Signal1/Subsystem/Switch Case Action Subsystem ==
  In1 : Inport
  Left_type : Inport  Port=2
  Action Port : ActionPort
  Bus Creator : BusCreator  Inputs=2
  Out1 : Outport
  wires:
  In1/1 -> Bus Creator/1  "A0"
  Left_type/1 -> Bus Creator/2  "Type"
  Bus Creator/1 -> Out1/1

== system PvtSubSys_HMI/HMI2.12/IFC_Signal1/Subsystem/Switch Case Action Subsystem1 ==
  In1 : Inport
  Action Port : ActionPort
  Bus Creator : BusCreator  Inputs=2
  Constant2 : Constant  Value=3  OutDataTypeStr=uint8
  Out1 : Outport
  wires:
  In1/1 -> Bus Creator/1  "A0"
  Bus Creator/1 -> Out1/1
  Constant2/1 -> Bus Creator/2  "Type"

== system PvtSubSys_HMI/HMI2.12/IFC_Signal1/Subsystem/Switch Case Action Subsystem2 ==
  In1 : Inport
  In2 : Inport  Port=2
  Action Port : ActionPort
  Bus Creator : BusCreator  Inputs=2
  Out1 : Outport
  wires:
  In1/1 -> Bus Creator/1  "A0"
  Bus Creator/1 -> Out1/1
  In2/1 -> Bus Creator/2  "Type"

== system PvtSubSys_HMI/HMI2.12/IFC_Signal1/Subsystem/Switch Case Action Subsystem3 ==
  In1 : Inport
  Action Port : ActionPort
  Bus Creator : BusCreator  Inputs=2
  Constant2 : Constant  Value=3  OutDataTypeStr=uint8
  Out1 : Outport
  wires:
  In1/1 -> Bus Creator/1  "A0"
  Bus Creator/1 -> Out1/1
  Constant2/1 -> Bus Creator/2  "Type"

== system PvtSubSys_HMI/HMI2.12/IFC_Signal1/Subsystem/Switch Case Action Subsystem4 ==
  Action Port : ActionPort
  Bus Creator : BusCreator  Inputs=2
  Constant1 : Constant  Value=0  OutDataTypeStr=single
  Constant2 : Constant  Value=0  OutDataTypeStr=uint8
  Out1 : Outport
  wires:
  Constant1/1 -> Bus Creator/1  "A0"
  Bus Creator/1 -> Out1/1
  Constant2/1 -> Bus Creator/2  "Type"

== system PvtSubSys_HMI/HMI2.12/IFC_Signal1/Subsystem/Switch Case Action Subsystem5 ==
  Action Port : ActionPort
  Bus Creator : BusCreator  Inputs=2
  Constant1 : Constant  Value=0  OutDataTypeStr=single
  Constant2 : Constant  Value=0  OutDataTypeStr=uint8
  Out1 : Outport
  wires:
  Constant1/1 -> Bus Creator/1  "A0"
  Constant2/1 -> Bus Creator/2  "Type"
  Bus Creator/1 -> Out1/1

== system PvtSubSys_HMI/HMI2.12/IFC_Signal1/Subsystem1/Switch Case Action Subsystem ==
  In1 : Inport
  In2 : Inport  Port=2
  A2 : Inport  Port=3
  A3 : Inport  Port=4
  Left_type : Inport  Port=5
  L_Valid : Inport  Port=6
  Action Port : ActionPort
  Bus Creator : BusCreator  Inputs=6
  Out1 : Outport
  wires:
  L_Valid/1 -> Bus Creator/6  "Valid"
  A3/1 -> Bus Creator/4  "A3"
  A2/1 -> Bus Creator/3  "A2"
  In2/1 -> Bus Creator/2  "A1"
  In1/1 -> Bus Creator/1  "A0"
  Left_type/1 -> Bus Creator/5  "Type"
  Bus Creator/1 -> Out1/1

== system PvtSubSys_HMI/HMI2.12/IFC_Signal1/Subsystem1/Switch Case Action Subsystem1 ==
  A0 : Inport
  A1 : Inport  Port=2
  A2 : Inport  Port=3
  A3 : Inport  Port=4
  LRE_Valid : Inport  Port=5
  Action Port : ActionPort
  Bus Creator1 : BusCreator  Inputs=6
  Constant : Constant  Value=3  OutDataTypeStr=uint8
  Out2 : Outport
  wires:
  LRE_Valid/1 -> Bus Creator1/6  "Valid"
  A1/1 -> Bus Creator1/2  "A1"
  Bus Creator1/1 -> Out2/1
  A2/1 -> Bus Creator1/3  "A2"
  A3/1 -> Bus Creator1/4  "A3"
  Constant/1 -> Bus Creator1/5  "Type"
  A0/1 -> Bus Creator1/1  "A0"

== system PvtSubSys_HMI/HMI2.12/IFC_Signal1/Subsystem1/Switch Case Action Subsystem2 ==
  A0 : Inport
  A1 : Inport  Port=2
  A2 : Inport  Port=3
  A3 : Inport  Port=4
  Right_type : Inport  Port=5
  Valid : Inport  Port=6
  Action Port : ActionPort
  Bus Creator : BusCreator  Inputs=6
  Out1 : Outport
  wires:
  Valid/1 -> Bus Creator/6  "Valid"
  A1/1 -> Bus Creator/2  "A1"
  Bus Creator/1 -> Out1/1
  A2/1 -> Bus Creator/3  "A2"
  A3/1 -> Bus Creator/4  "A3"
  Right_type/1 -> Bus Creator/5  "Type"
  A0/1 -> Bus Creator/1  "A0"

== system PvtSubSys_HMI/HMI2.12/IFC_Signal1/Subsystem1/Switch Case Action Subsystem3 ==
  A0 : Inport
  A1 : Inport  Port=2
  A2 : Inport  Port=3
  A3 : Inport  Port=4
  Valid : Inport  Port=5
  Action Port : ActionPort
  Bus Creator : BusCreator  Inputs=6
  Constant : Constant  Value=3  OutDataTypeStr=uint8
  Out1 : Outport
  wires:
  Valid/1 -> Bus Creator/6  "Valid"
  A1/1 -> Bus Creator/2  "A1"
  Bus Creator/1 -> Out1/1
  A2/1 -> Bus Creator/3  "A2"
  A3/1 -> Bus Creator/4  "A3"
  Constant/1 -> Bus Creator/5  "Type"
  A0/1 -> Bus Creator/1  "A0"

== system PvtSubSys_HMI/HMI2.12/IFC_Signal1/Subsystem1/Switch Case Action Subsystem4 ==
  Action Port : ActionPort
  Bus Creator1 : BusCreator  Inputs=6
  Constant{,1..3} (4 alike) : Constant  Value=0  OutDataTypeStr=single
  Constant4 : Constant  Value=0  OutDataTypeStr=uint8
  Constant6 : Constant  OutDataTypeStr=uint8
  Out2 : Outport
  wires:
  Constant6/1 -> Bus Creator1/6  "Valid"
  Constant1/1 -> Bus Creator1/2  "A1"
  Bus Creator1/1 -> Out2/1
  Constant2/1 -> Bus Creator1/3  "A2"
  Constant3/1 -> Bus Creator1/4  "A3"
  Constant4/1 -> Bus Creator1/5  "Type"
  Constant/1 -> Bus Creator1/1  "A0"

== system PvtSubSys_HMI/HMI2.12/IFC_Signal1/Subsystem1/Switch Case Action Subsystem5 ==
  Action Port : ActionPort
  Bus Creator : BusCreator  Inputs=6
  Constant{1,3..5} (4 alike) : Constant  Value=0  OutDataTypeStr=single
  Constant2 : Constant  Value=0  OutDataTypeStr=uint8
  Constant7 : Constant  OutDataTypeStr=uint8
  Out1 : Outport
  wires:
  Constant7/1 -> Bus Creator/6  "Valid"
  Constant5/1 -> Bus Creator/4  "A3"
  Constant4/1 -> Bus Creator/3  "A2"
  Constant3/1 -> Bus Creator/2  "A1"
  Constant1/1 -> Bus Creator/1  "A0"
  Constant2/1 -> Bus Creator/5  "Type"
  Bus Creator/1 -> Out1/1

== system PvtSubSys_HMI/HMI2.12/IFC_Signal1/Subsystem2/Switch Case Action Subsystem ==
  In1 : Inport
  Left_type : Inport  Port=2
  Action Port : ActionPort
  Bus Creator : BusCreator  Inputs=2
  Out1 : Outport
  wires:
  Bus Creator/1 -> Out1/1
  Left_type/1 -> Bus Creator/2  "Type"
  In1/1 -> Bus Creator/1  "A0"

== system PvtSubSys_HMI/HMI2.12/IFC_Signal1/Subsystem2/Switch Case Action Subsystem1 ==
  In1 : Inport
  Action Port : ActionPort
  Bus Creator : BusCreator  Inputs=2
  Constant2 : Constant  Value=3  OutDataTypeStr=uint8
  Out1 : Outport
  wires:
  Constant2/1 -> Bus Creator/2  "Type"
  Bus Creator/1 -> Out1/1
  In1/1 -> Bus Creator/1  "A0"

== system PvtSubSys_HMI/HMI2.12/IFC_Signal1/Subsystem2/Switch Case Action Subsystem2 ==
  In1 : Inport
  In2 : Inport  Port=2
  Action Port : ActionPort
  Bus Creator : BusCreator  Inputs=2
  Out1 : Outport
  wires:
  In2/1 -> Bus Creator/2  "Type"
  Bus Creator/1 -> Out1/1
  In1/1 -> Bus Creator/1  "A0"

== system PvtSubSys_HMI/HMI2.12/IFC_Signal1/Subsystem2/Switch Case Action Subsystem3 ==
  In1 : Inport
  Action Port : ActionPort
  Bus Creator : BusCreator  Inputs=2
  Constant2 : Constant  Value=3  OutDataTypeStr=uint8
  Out1 : Outport
  wires:
  Constant2/1 -> Bus Creator/2  "Type"
  Bus Creator/1 -> Out1/1
  In1/1 -> Bus Creator/1  "A0"

== system PvtSubSys_HMI/HMI2.12/IFC_Signal1/Subsystem2/Switch Case Action Subsystem4 ==
  Action Port : ActionPort
  Bus Creator : BusCreator  Inputs=2
  Constant1 : Constant  Value=0  OutDataTypeStr=single
  Constant2 : Constant  Value=0  OutDataTypeStr=uint8
  Out1 : Outport
  wires:
  Constant2/1 -> Bus Creator/2  "Type"
  Bus Creator/1 -> Out1/1
  Constant1/1 -> Bus Creator/1  "A0"

== system PvtSubSys_HMI/HMI2.12/IFC_Signal1/Subsystem2/Switch Case Action Subsystem5 ==
  Action Port : ActionPort
  Bus Creator : BusCreator  Inputs=2
  Constant1 : Constant  Value=0  OutDataTypeStr=single
  Constant2 : Constant  Value=0  OutDataTypeStr=uint8
  Out1 : Outport
  wires:
  Bus Creator/1 -> Out1/1
  Constant2/1 -> Bus Creator/2  "Type"
  Constant1/1 -> Bus Creator/1  "A0"

== matlab function PvtSubSys_HMI/HMI2.12/HWA//ACC//TJA_Signal1/MATLAB Function5 ==
  data: AngRaw input single; Angle output single
function Angle = AngCalc(AngRaw)
if AngRaw>1.57
    Angle = AngRaw - single(3.14);
elseif AngRaw<-1.57
    Angle = AngRaw + single(3.14);
else
    Angle = AngRaw;
end

== matlab function PvtSubSys_HMI/HMI2.12/HWA//ACC//TJA_Signal1/MATLAB Function6 ==
  data: AngRaw input single; Angle output single
function Angle = AngCalc(AngRaw)
if AngRaw>1.57
    Angle = AngRaw - single(3.14);
elseif AngRaw<-1.57
    Angle = AngRaw + single(3.14);
else
    Angle = AngRaw;
end
